simulink model "SineWaveCommand"  (R2021a)
settings: Solver=VariableStepAuto  StartTime=0.0  StopTime=inf  RelTol=1e-3
undefined symbols (not defined in the file or in its folder): f
libraries: simulink x3, instrumentlib x3
settings Model: EnablePacing=on  Creator=vecluster  LastModifiedBy=LAR
settings DataIOCC: LoggingToFile=on  LoggingFileName=Test.mat

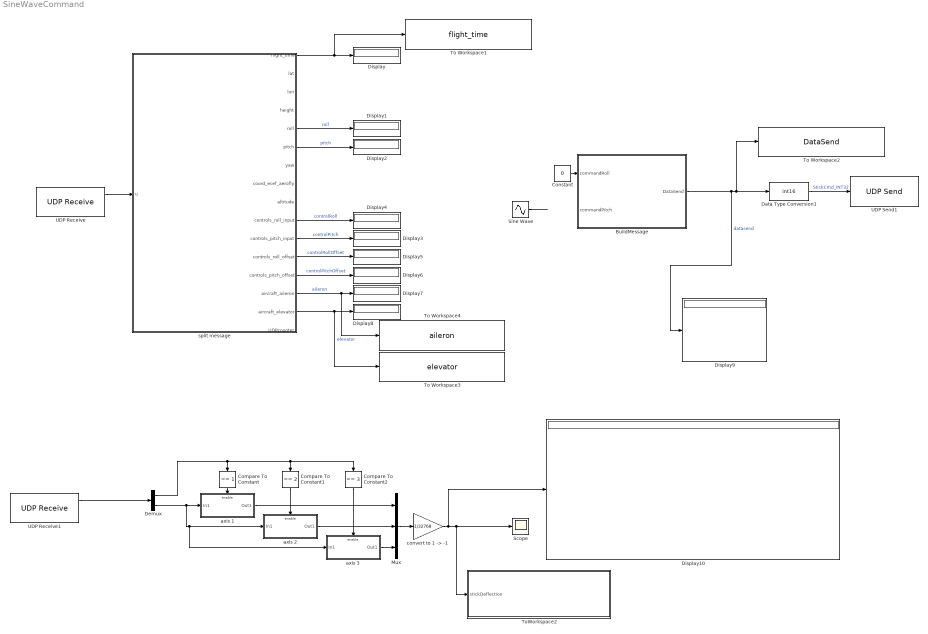
== system SineWaveCommand ==
  BuildMessage : MATLAB Function  TreatAsAtomicUnit=on
  Compare To Constant : simulink/Logic and Bit Operations/Compare To Constant  relop===  const=1  OutDataTypeStr=boolean
  Compare To Constant1 : simulink/Logic and Bit Operations/Compare To Constant  relop===  const=2  OutDataTypeStr=boolean
  Compare To Constant2 : simulink/Logic and Bit Operations/Compare To Constant  relop===  const=3  OutDataTypeStr=boolean
  Constant : Constant  Value=0
  Data Type Conversion1 : DataTypeConversion  OutDataTypeStr=int16
  Demux : Demux  Outputs=2
  Display{,1..10} (11 alike) : Display
  Mux : Mux  Inputs=3
  Scope : Scope
  Sine Wave : Sin  Frequency=1000  SampleTime=0.01
  To Workspace1 : ToWorkspace  VariableName=flight_time  SaveFormat=Structure With Time  SampleTime=-1
  To Workspace2 : ToWorkspace  VariableName=DataSend  SaveFormat=Structure With Time  SampleTime=-1
  To Workspace3 : ToWorkspace  VariableName=elevator  SaveFormat=Structure With Time  SampleTime=-1
  To Workspace4 : ToWorkspace  VariableName=aileron  SaveFormat=Structure With Time  SampleTime=-1
  ToWorkspace2 : Subsystem
  UDP Receive : instrumentlib/UDP Receive  Host=0.0.0.0  Port=1  LocalPort=6060  EnablePortSharing=on  GetLatestData=on  DataSize="[20   1]"  DataType=double  ASCIIFormatting=%f,  Terminator=LF  ByteOrder=LittleEndian  EnableBlockingMode=off  Timeout=100  SampleTime=0.01  LocalAddress=127.0.0.1
  UDP Receive1 : instrumentlib/UDP Receive  Host=0.0.0.0  Port=1  LocalPort=15346  EnablePortSharing=on  GetLatestData=on  DataSize="[2  1]"  DataType=double  ASCIIFormatting=%f,  Terminator=LF  ByteOrder=LittleEndian  EnableBlockingMode=off  Timeout=100  SampleTime=0.01  LocalAddress=192.168.51.167
  UDP Send1 : instrumentlib/UDP Send  Host=192.168.51.103  Port=5347  LocalPort=-1  EnablePortSharing=on  ByteOrder=LittleEndian  OutputDatagramPacketSize=512  EnableBlockingMode=on  LocalAddress=0.0.0.0
  axis 1 : Subsystem  TreatAsAtomicUnit=on
  axis 2 : Subsystem  TreatAsAtomicUnit=on
  axis 3 : Subsystem  TreatAsAtomicUnit=on
  "convert to 1 -> -1" : Gain  Gain=1/32768
  split message : MATLAB Function  TreatAsAtomicUnit=on
  wires:
  Data Type Conversion1/1 -> UDP Send1/1  "StickCmd_INT32"
  split message/15(aircraft_elevator) -> To Workspace3/1, Display8/1  "elevator"
  UDP Receive/1 -> split message/1(u)
  split message/14(aircraft_aileron) -> To Workspace4/1, Display7/1  "aileron"
  split message/12(controls_roll_offset) -> Display5/1  "controlRollOffset"
  split message/11(controls_pitch_input) -> Display3/1  "controlPitch"
  split message/5(roll) -> Display1/1  "roll"
  split message/6(pitch) -> Display2/1  "pitch"
  split message/1(flight_time) -> To Workspace1/1, Display/1
  split message/13(controls_pitch_offset) -> Display6/1  "controlPitchOffset"
  split message/10(controls_roll_input) -> Display4/1  "controlRoll"
  BuildMessage/1(DataSend) -> Display9/1, To Workspace2/1, Data Type Conversion1/1  "datasend"
  Sine Wave/1 -> ?
  Constant/1 -> BuildMessage/1(commandRoll)
  Mux/1 -> "convert to 1 -> -1"/1
  axis 2/1(Out1) -> Mux/2
  Compare To Constant1/1 -> axis 2/Enable
  "convert to 1 -> -1"/1 -> Display10/1, ToWorkspace2/1(stickDeflection), Scope/1
  Compare To Constant/1 -> axis 1/Enable
  axis 1/1(Out1) -> Mux/1
  Compare To Constant2/1 -> axis 3/Enable
  Demux/1 -> Compare To Constant/1, Compare To Constant1/1, Compare To Constant2/1
  Demux/2 -> axis 3/1(In1), axis 2/1(In1), axis 1/1(In1)
  axis 3/1(Out1) -> Mux/3
  UDP Receive1/1 -> Demux/1

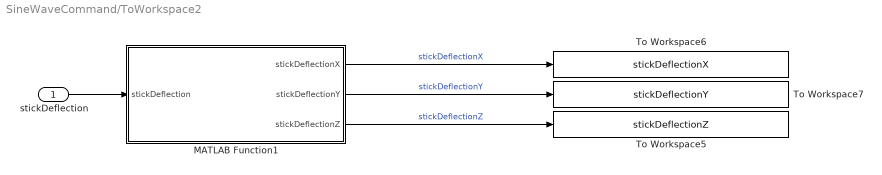
== system SineWaveCommand/ToWorkspace2 ==
  stickDeflection : Inport
  MATLAB Function1 : MATLAB Function  TreatAsAtomicUnit=on
  To Workspace5 : ToWorkspace  VariableName=stickDeflectionZ  SaveFormat=Structure With Time  SampleTime=-1
  To Workspace6 : ToWorkspace  VariableName=stickDeflectionX  SaveFormat=Structure With Time  SampleTime=-1
  To Workspace7 : ToWorkspace  VariableName=stickDeflectionY  SaveFormat=Structure With Time  SampleTime=-1
  wires:
  MATLAB Function1/2(stickDeflectionY) -> To Workspace7/1  "stickDeflectionY"
  MATLAB Function1/3(stickDeflectionZ) -> To Workspace5/1  "stickDeflectionZ"
  MATLAB Function1/1(stickDeflectionX) -> To Workspace6/1  "stickDeflectionX"
  stickDeflection/1 -> MATLAB Function1/1(stickDeflection)

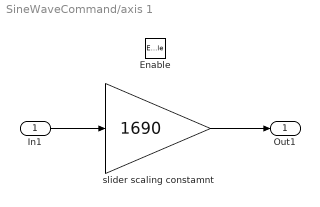
== system SineWaveCommand/axis 1 ==
  In1 : Inport
  Enable : EnablePort
  slider scaling constamnt : Gain  Gain=1690
  Out1 : Outport
  wires:
  In1/1 -> slider scaling constamnt/1
  slider scaling constamnt/1 -> Out1/1

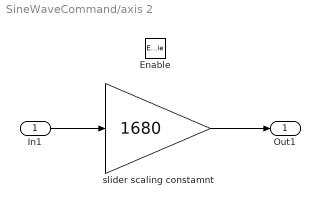
== system SineWaveCommand/axis 2 ==
  In1 : Inport
  Enable : EnablePort
  slider scaling constamnt : Gain  Gain=1680
  Out1 : Outport
  wires:
  In1/1 -> slider scaling constamnt/1
  slider scaling constamnt/1 -> Out1/1

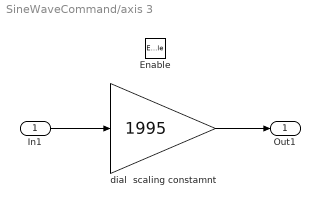
== system SineWaveCommand/axis 3 ==
  In1 : Inport
  Enable : EnablePort
  dial  scaling constamnt : Gain  Gain=1995
  Out1 : Outport
  wires:
  In1/1 -> dial  scaling constamnt/1
  dial  scaling constamnt/1 -> Out1/1

== matlab function SineWaveCommand/split message ==
  data: u input; flight_time output; lat output; lon output; height output; roll output; pitch output; yaw output; coord_ecef_aerofly output; altitude output; controls_roll_input output; controls_pitch_input output; controls_roll_offset output; controls_pitch_offset output; aircraft_aileron output; aircraft_elevator output; UDPcounter output
function [flight_time, lat, lon, height, roll, pitch, yaw, ...
          coord_ecef_aerofly, altitude,  controls_roll_input,...
          controls_pitch_input, controls_roll_offset, controls_pitch_offset, aircraft_aileron, aircraft_elevator, UDPcounter] = split(u)
 
%// send binary data to matlab
% 	gAircraftData2MatlabBuffer[0] = lfFlightTimeS;
% 
% 	gAircraftData2MatlabBuffer[1] = aircraft_position.x;
% 	gAircraftData2MatlabBuffer[2] = aircraft_position.y;
% 	gAircraftData2MatlabBuffer[3] = aircraft_position.z;
% 
% 	gAircraftData2MatlabBuffer[4] = aircraft_latitude;
% 	gAircraftData2MatlabBuffer[5] = aircraft_longitude;
% 
% 	gAircraftData2MatlabBuffer[6] = aircraft_height;
% 
% 	gAircraftData2MatlabBuffer[7] = aircraft_altitude;
% 
% 	gAircraftData2MatlabBuffer[8] = aircraft_bank;
% 	gAircraftData2MatlabBuffer[9] = aircraft_pitch;
% 	gAircraftData2MatlabBuffer[10] = aircraft_heading;
% 	gAircraftData2MatlabBuffer[11] = controls_roll_input;
% 	gAircraftData2MatlabBuffer[12] = controls_pitch_input;
% 	gAircraftData2MatlabBuffer[13] = controls_yaw_input;
% 	gAircraftData2MatlabBuffer[14] = controls_roll_input_offset;
% 	gAircraftData2MatlabBuffer[15] = controls_pitch_input_offset;
%   gAircraftData2MatlabBuffer[16] = aircraft_aileron;
%   gAircraftData2MatlabBuffer[17] = aircraft_elevator;
	
% 
% 	// ...
% 	gAircraftData2MatlabBuffer[19] = nUdpCounter;



    flight_time = u(1);
    x_pos = u(2);
    y_pos = u(3);
    z_pos = - u(4);
    coord_ecef_aerofly = [x_pos, y_pos, - z_pos];
    
    lat = u(5);
    lon = u(6);
    height = u(7);
    
    altitude = u(8);
    
    roll = rad2deg(u(9));
    pitch = rad2deg(u(10));
    %pay attention the conversion is made just here and not in the logfile
    %this way the angle will be referred to the north and counted clockwise
    %for now we don't use it, but pay attention to the local frame and the
    %reference systems of the other angles if using them together for the
    %feedback
    yaw = 360 - rad2deg(u(11)) + 90;
    
    controls_roll_input = u(10); %rad2deg(u(10));
    controls_pitch_input = u(11); %rad2deg(u(11));
    
    controls_roll_offset = u(13); % rad2deg(u(13));
    controls_pitch_offset = u(14); %rad2deg(u(14));
    
    aircraft_aileron = u(15); 
    aircraft_elevator = u(16); 
    
    
    UDPcounter = u(20);
    
    
end

== matlab function SineWaveCommand/BuildMessage ==
  data: commandRoll input; DataSend output; commandPitch input
function DataSend = fcn(commandRoll,commandPitch)
    DataSend = zeros(1,12);
    
    %test sinus
%     amplitude = 32000;
%     x = 0:0.1:20*pi;
%     y = sin(frequency*x)*amplitude;
    
    %spring
    springRoll = 500;
    springPitch = 450;
    
    %friction 
    frictionRoll = 0;
    frictionPitch = 0;
    
    %damping 
    dampingRoll = 0;
    dampingPitch = 0;
    
    %torque    
    torqueRoll = 700*commandRoll;
    torquePitch = 750*commandPitch;

    %Build DataSend
    DataSend(1) = springRoll;
    DataSend(2) = frictionRoll;
    DataSend(3) = dampingRoll;
    DataSend(4) = torqueRoll;
    
    DataSend(5) = springPitch;
    DataSend(6) = frictionPitch;
    DataSend(7) = dampingPitch;
    DataSend(8) = torquePitch;

== matlab function SineWaveCommand/ToWorkspace2/MATLAB Function1 ==
  data: stickDeflection input; stickDeflectionX output; stickDeflectionY output; stickDeflectionZ output
function [stickDeflectionX, stickDeflectionY, stickDeflectionZ] = split(stickDeflection)
          stickDeflectionX = stickDeflection(1);
          stickDeflectionY = stickDeflection(2);
          stickDeflectionZ = stickDeflection(3);
